simulink model "gm_uz_dac_spi_interface"  (R2023a)
settings: Solver=FixedStepDiscrete  StartTime=0.0  StopTime=2000/100e6  RelTol=1e-3
libraries: hdlsllib x152, simulink x3
settings Model: Creator=ts  LastModifiedBy=ts
settings SolverCC: AlgebraicLoopSolver=TrustRegion
settings DataIOCC: LimitDataPoints=on  SaveOutput=off  SaveTime=off
settings OptimizationCC: BlockReduction=off  ConditionallyExecuteInputs=off  DefaultParameterBehavior=Inlined  LifeSpan=inf
settings DebuggingCC: AlgebraicLoopMsg=error  InheritedTsInSrcMsg=none  SingleTaskRateTransMsg=error  UnconnectedInputMsg=warning  UnconnectedOutputMsg=warning  UnconnectedLineMsg=warning  AllowSymbolicDim=off  StrictBusMsg=ErrorOnBusTreatedAsVector  SFUnexpectedBacktrackingDiag=warning  SFNoUnconditionalDefaultTransitionDiag=warning  SFExecutionAtInitializationDiag=none  ArithmeticOperatorsInVariantConditions=warning
settings HardwareCC: ProdBitPerPointer=32  ProdBitPerSizeT=32  ProdBitPerPtrDiffT=32  ProdLargestAtomicFloat=None  ProdIntDivRoundTo=Undefined  ProdEndianess=Unspecified  ProdWordSize=32  ProdHWDeviceType=ASIC/FPGA->ASIC/FPGA  ProdEqTarget=off
settings ModelReferenceCC: EnableRefExpFcnMdlSchedulingChecks=on
settings SFSimCC: SimUseLocalCustomCode=off  CustomCodeUndefinedFunction=UseInterfaceOnly
settings RTWCC: RTWUseLocalCustomCode=off
settings CodeAppCC: StateflowObjectComments=on
settings GRTTargetCC: TargetLangStandard=C89/C90 (ANSI)
settings ConfigComp: CovScope=ReferencedModels  CovMetricSettings=dw  CovSaveCumulativeToWorkspaceVar=on  CovSaveSingleToWorkspaceVar=on  CovExternalEMLEnable=off  CovSFcnEnable=off

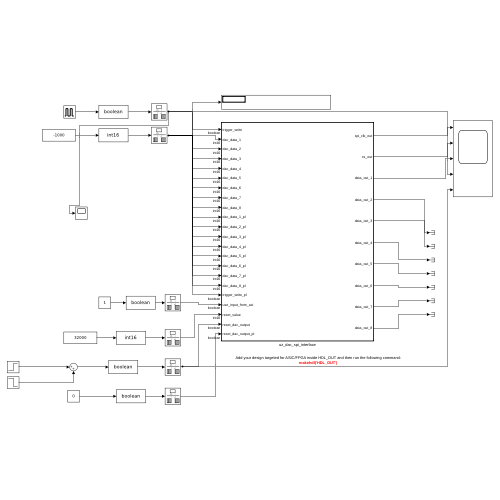
[thumbnail: Simulink's stored preview of the top-level diagram]
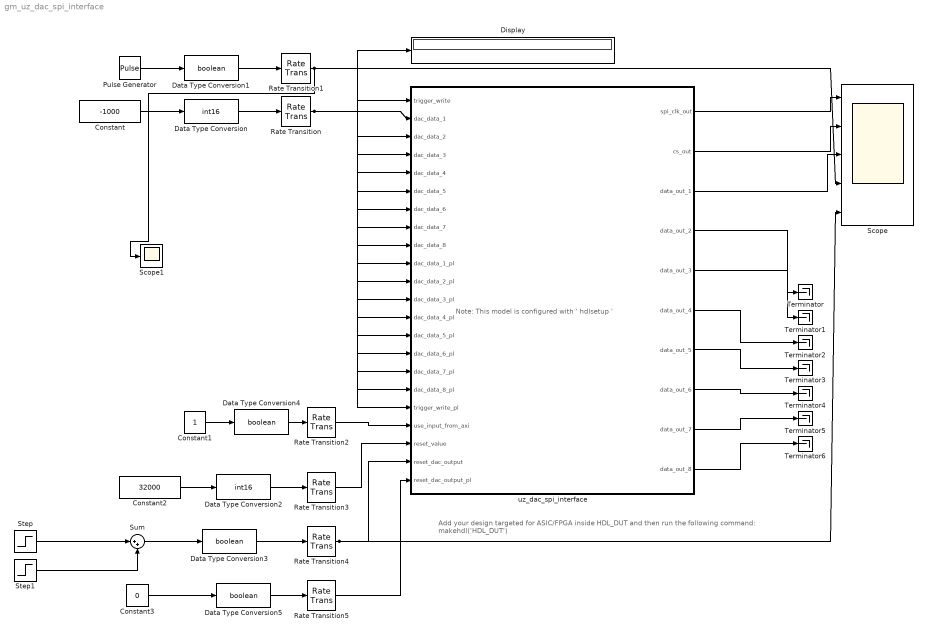
== system gm_uz_dac_spi_interface ==
  note: Add your design targeted for ASIC/FPGA inside HDL_DUT and then run the following command:
      | makehdl('HDL_DUT')
  note: Note: This model is configured with ' hdlsetup '
  Constant : Constant  Value=-1000  OutDataTypeStr=int16  SampleTime=1/100e6
  Constant1 : Constant
  Constant2 : Constant  Value=32000  OutDataTypeStr=int16  SampleTime=1/100e6
  Constant3 : Constant  Value=0
  Data Type Conversion : DataTypeConversion  OutDataTypeStr=int16  SaturateOnIntegerOverflow=off  RndMeth=Floor
  Data Type Conversion{1,3..5} (4 alike) : DataTypeConversion  OutDataTypeStr=boolean  SaturateOnIntegerOverflow=off  RndMeth=Floor
  Data Type Conversion2 : DataTypeConversion  OutDataTypeStr=int16  SaturateOnIntegerOverflow=off  RndMeth=Floor
  Display : Display
      settings: Format=binary (Stored Integer)
  Pulse Generator : DiscretePulseGenerator  PulseType=Time based  Period=200/100e6  PulseWidth=10
  Rate Transition{,1..5} (6 alike) : RateTransition  OutPortSampleTime=1/100e6
  Scope : Scope  NumInputPorts=5
  Scope1 : Scope
  Step : Step  Time=280/100e6  SampleTime=1/100e6  VectorParams1D=off
  Step1 : Step  Time=800/100e6  After=-1  SampleTime=1/100e6
  Sum : Sum  Inputs=|++
  Terminator{,1..6} (7 alike) : Terminator
  uz_dac_spi_interface : Subsystem  TreatAsAtomicUnit=on
  wires:
  Sum/1 -> Data Type Conversion3/1
  Step1/1 -> Sum/2
  Step/1 -> Sum/1
  Rate Transition4/1 -> uz_dac_spi_interface/21(reset_dac_output), Scope/5
  Data Type Conversion5/1 -> Rate Transition5/1
  Data Type Conversion4/1 -> Rate Transition2/1
  Rate Transition5/1 -> uz_dac_spi_interface/22(reset_dac_output_pl)
  Constant3/1 -> Data Type Conversion5/1
  Data Type Conversion3/1 -> Rate Transition4/1
  Rate Transition3/1 -> uz_dac_spi_interface/20(reset_value)
  Data Type Conversion2/1 -> Rate Transition3/1
  Constant2/1 -> Data Type Conversion2/1
  uz_dac_spi_interface/10(data_out_8) -> Terminator6/1
  uz_dac_spi_interface/9(data_out_7) -> Terminator5/1
  uz_dac_spi_interface/8(data_out_6) -> Terminator4/1
  uz_dac_spi_interface/7(data_out_5) -> Terminator3/1
  uz_dac_spi_interface/6(data_out_4) -> Terminator2/1
  uz_dac_spi_interface/5(data_out_3) -> Terminator1/1
  uz_dac_spi_interface/4(data_out_2) -> Terminator/1
  Constant1/1 -> Data Type Conversion4/1
  Rate Transition2/1 -> uz_dac_spi_interface/19(use_input_from_axi)
  Pulse Generator/1 -> Data Type Conversion1/1
  Data Type Conversion1/1 -> Rate Transition1/1
  Rate Transition1/1 -> Scope1/1, uz_dac_spi_interface/18(trigger_write_pl), uz_dac_spi_interface/1(trigger_write), Scope/4
  uz_dac_spi_interface/1(spi_clk_out) -> Scope/1
  uz_dac_spi_interface/2(cs_out) -> Scope/2
  Rate Transition/1 -> uz_dac_spi_interface/2(dac_data_1), uz_dac_spi_interface/3(dac_data_2), uz_dac_spi_interface/4(dac_data_3), uz_dac_spi_interface/5(dac_data_4), uz_dac_spi_interface/6(dac_data_5), uz_dac_spi_interface/8(dac_data_7), uz_dac_spi_interface/9(dac_data_8), uz_dac_spi_interface/10(dac_data_1_pl), uz_dac_spi_interface/11(dac_data_2_pl), uz_dac_spi_interface/12(dac_data_3_pl), uz_dac_spi_interface/13(dac_data_4_pl), uz_dac_spi_interface/14(dac_data_5_pl), uz_dac_spi_interface/15(dac_data_6_pl), uz_dac_spi_interface/16(dac_data_7_pl), uz_dac_spi_interface/17(dac_data_8_pl), uz_dac_spi_interface/7(dac_data_6), Display/1
  Data Type Conversion/1 -> Rate Transition/1
  uz_dac_spi_interface/3(data_out_1) -> Scope/3
  Constant/1 -> Data Type Conversion/1

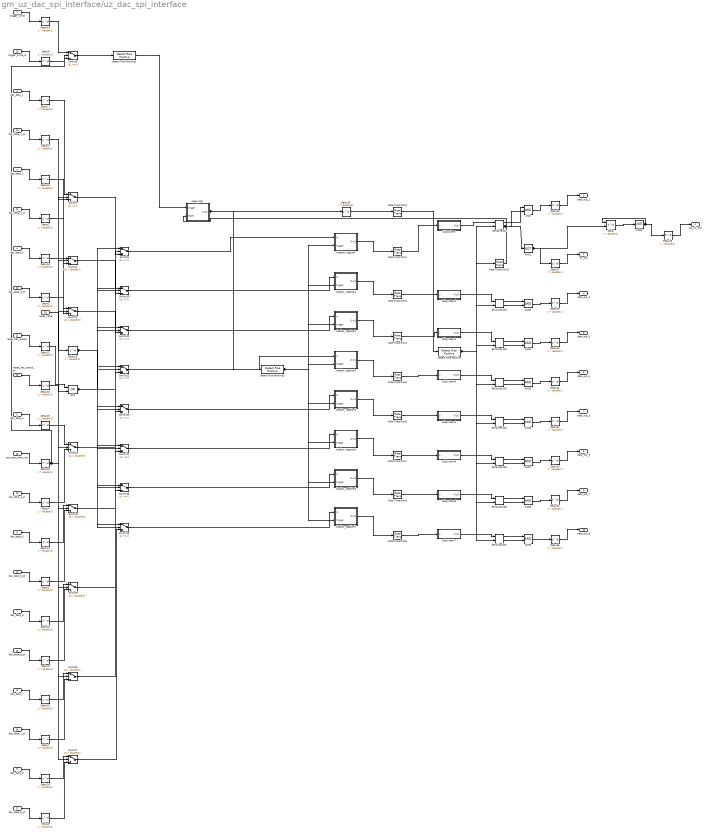
== system gm_uz_dac_spi_interface/uz_dac_spi_interface ==
  trigger_write : Inport  OutDataTypeStr=boolean  PortDimensions=1  SampleTime=1e-08
  dac_data_1 : Inport  Port=2  OutDataTypeStr=int16  PortDimensions=1  SampleTime=1e-08
  dac_data_2 : Inport  Port=3  OutDataTypeStr=int16  PortDimensions=1  SampleTime=1e-08
  dac_data_3 : Inport  Port=4  OutDataTypeStr=int16  PortDimensions=1  SampleTime=1e-08
  dac_data_4 : Inport  Port=5  OutDataTypeStr=int16  PortDimensions=1  SampleTime=1e-08
  dac_data_5 : Inport  Port=6  OutDataTypeStr=int16  PortDimensions=1  SampleTime=1e-08
  dac_data_6 : Inport  Port=7  OutDataTypeStr=int16  PortDimensions=1  SampleTime=1e-08
  dac_data_7 : Inport  Port=8  OutDataTypeStr=int16  PortDimensions=1  SampleTime=1e-08
  dac_data_8 : Inport  Port=9  OutDataTypeStr=int16  PortDimensions=1  SampleTime=1e-08
  dac_data_1_pl : Inport  Port=10  OutDataTypeStr=int16  PortDimensions=1  SampleTime=1e-08
  dac_data_2_pl : Inport  Port=11  OutDataTypeStr=int16  PortDimensions=1  SampleTime=1e-08
  dac_data_3_pl : Inport  Port=12  OutDataTypeStr=int16  PortDimensions=1  SampleTime=1e-08
  dac_data_4_pl : Inport  Port=13  OutDataTypeStr=int16  PortDimensions=1  SampleTime=1e-08
  dac_data_5_pl : Inport  Port=14  OutDataTypeStr=int16  PortDimensions=1  SampleTime=1e-08
  dac_data_6_pl : Inport  Port=15  OutDataTypeStr=int16  PortDimensions=1  SampleTime=1e-08
  dac_data_7_pl : Inport  Port=16  OutDataTypeStr=int16  PortDimensions=1  SampleTime=1e-08
  dac_data_8_pl : Inport  Port=17  OutDataTypeStr=int16  PortDimensions=1  SampleTime=1e-08
  trigger_write_pl : Inport  Port=18  OutDataTypeStr=boolean  PortDimensions=1  SampleTime=1e-08
  use_input_from_axi : Inport  Port=19  OutDataTypeStr=boolean  PortDimensions=1  SampleTime=1e-08
  reset_value : Inport  Port=20  OutDataTypeStr=int16  PortDimensions=1  SampleTime=1e-08
  reset_dac_output : Inport  Port=21  OutDataTypeStr=boolean  PortDimensions=1  SampleTime=1e-08
  reset_dac_output_pl : Inport  Port=22  OutDataTypeStr=boolean  PortDimensions=1  SampleTime=1e-08
  AND{,3..9} (8 alike) : Logic  AllPortsSameDT=off  OutDataTypeStr=boolean  SampleTime=1e-08
  AND1 : Logic  Operator=NOT  Inputs=1  AllPortsSameDT=off  OutDataTypeStr=boolean  SampleTime=1e-08
  AND2 : Logic  Operator=NOT  Inputs=1  AllPortsSameDT=off  OutDataTypeStr=boolean  SampleTime=1e-08
  Delay : Delay  DelayLength=double(1)  InitialCondition=1  ExternalReset=Level
      settings: InputPortMap=u0,r5
  Delay{1..10,12..15,17..35} (33 alike) : Delay  DelayLength=double(1)  InitialCondition=0  SampleTime=1e-08
  Detect Rise Positive : simulink/Logic and Bit Operations/Detect Rise Positive  vinit=0  OutDataTypeStr=boolean
  Detect Rise Positive1 : simulink/Logic and Bit Operations/Detect Rise Positive  vinit=0  OutDataTypeStr=boolean
  Detect Rise Positive2 : simulink/Logic and Bit Operations/Detect Rise Positive  vinit=0  OutDataTypeStr=boolean
  OR1 : Logic  Operator=OR  AllPortsSameDT=off  OutDataTypeStr=boolean  SampleTime=1e-08
  Rate Transition{1..9} (9 alike) : RateTransition  InitialCondition=double(0)  OutPortSampleTimeOpt=Multiple of input port sample time  OutPortSampleTimeMultiple=32
  Rate Transition11 : RateTransition  InitialCondition=double(0)  OutPortSampleTimeOpt=Multiple of input port sample time  OutPortSampleTimeMultiple=1/32
  Serializer1D{,1..7} (8 alike) : hdlsllib/HDL Operations/Serializer1D  Ratio=32  IdleCycles=0  validIn=on  startOut=off  validOut=on  inputDataDimensions=32  inputSampleTime=3.2e-07  inputSignalType=real
  Subsystem : Subsystem
  Subsystem1 : Subsystem
  Subsystem2 : Subsystem
  Subsystem3 : Subsystem
  Subsystem4 : Subsystem
  Subsystem5 : Subsystem
  Subsystem6 : Subsystem
  Subsystem7 : Subsystem
  Switch{,9..16} (9 alike) : Switch  Criteria=u2 ~= 0  Threshold=double(0)  OutDataTypeStr=int16  SampleTime=1e-08  SaturateOnIntegerOverflow=off  InputSameDT=off
  Switch{1..7} (7 alike) : Switch  Criteria=u2 > Threshold  Threshold=double(0)  OutDataTypeStr=int16  SampleTime=1e-08  SaturateOnIntegerOverflow=off  InputSameDT=off
  Switch8 : Switch  Criteria=u2 ~= 0  Threshold=double(0)  OutDataTypeStr=boolean  SampleTime=1e-08  SaturateOnIntegerOverflow=off  InputSameDT=off
  keep_high : Subsystem
  shadow_register : Subsystem
  shadow_register1 : Subsystem
  shadow_register2 : Subsystem
  shadow_register3 : Subsystem
  shadow_register4 : Subsystem
  shadow_register5 : Subsystem
  shadow_register6 : Subsystem
  shadow_register7 : Subsystem
  spi_clk_out : Outport  SampleTime=1e-08
  cs_out : Outport  Port=2  SampleTime=1e-08
  data_out_1 : Outport  Port=3  SampleTime=1e-08  VectorParamsAs1DForOutWhenUnconnected=off
  data_out_2 : Outport  Port=4  SampleTime=1e-08  VectorParamsAs1DForOutWhenUnconnected=off
  data_out_3 : Outport  Port=5  SampleTime=1e-08  VectorParamsAs1DForOutWhenUnconnected=off
  data_out_4 : Outport  Port=6  SampleTime=1e-08  VectorParamsAs1DForOutWhenUnconnected=off
  data_out_5 : Outport  Port=7  SampleTime=1e-08  VectorParamsAs1DForOutWhenUnconnected=off
  data_out_6 : Outport  Port=8  SampleTime=1e-08  VectorParamsAs1DForOutWhenUnconnected=off
  data_out_7 : Outport  Port=9  SampleTime=1e-08  VectorParamsAs1DForOutWhenUnconnected=off
  data_out_8 : Outport  Port=10  SampleTime=1e-08  VectorParamsAs1DForOutWhenUnconnected=off
  wires:
  trigger_write/1 -> Delay14/1
  dac_data_1/1 -> Delay17/1
  dac_data_2/1 -> Delay19/1
  dac_data_3/1 -> Delay18/1
  dac_data_4/1 -> Delay20/1
  dac_data_5/1 -> Delay21/1
  dac_data_6/1 -> Delay22/1
  dac_data_7/1 -> Delay23/1
  dac_data_8/1 -> Delay24/1
  dac_data_1_pl/1 -> Delay1/1
  dac_data_2_pl/1 -> Delay2/1
  dac_data_3_pl/1 -> Delay3/1
  dac_data_4_pl/1 -> Delay4/1
  dac_data_5_pl/1 -> Delay5/1
  dac_data_6_pl/1 -> Delay6/1
  dac_data_7_pl/1 -> Delay7/1
  dac_data_8_pl/1 -> Delay8/1
  trigger_write_pl/1 -> Delay9/1
  use_input_from_axi/1 -> Delay15/1
  reset_value/1 -> Delay13/1
  reset_dac_output/1 -> Delay12/1
  reset_dac_output_pl/1 -> Delay10/1
  AND/1 -> Delay28/1
  AND1/1 -> Delay27/1, Delay/2
  AND2/1 -> Delay26/1, Delay/1
  AND3/1 -> Delay29/1
  AND4/1 -> Delay30/1
  AND5/1 -> Delay31/1
  AND6/1 -> Delay32/1
  AND7/1 -> Delay33/1
  AND8/1 -> Delay34/1
  AND9/1 -> Delay35/1
  Delay/1 -> AND2/1
  Delay1/1 -> Switch/3
  Delay10/1 -> OR1/2
  Delay12/1 -> OR1/1
  Delay13/1 -> Switch9/1, Switch16/1, Switch15/1, Switch14/1, Switch13/1, Switch12/1, Switch11/1, Switch10/1
  Delay14/1 -> Switch8/1
  Delay15/1 -> Switch8/2, Switch7/2, Switch6/2, Switch5/2, Switch4/2, Switch3/2, Switch2/2, Switch1/2, Switch/2
  Delay17/1 -> Switch/1
  Delay18/1 -> Switch2/1
  Delay19/1 -> Switch1/1
  Delay2/1 -> Switch1/3
  Delay20/1 -> Switch3/1
  Delay21/1 -> Switch4/1
  Delay22/1 -> Switch5/1
  Delay23/1 -> Switch6/1
  Delay24/1 -> Switch7/1
  Delay25/1 -> Rate Transition2/1
  Delay26/1 -> spi_clk_out/1
  Delay27/1 -> cs_out/1
  Delay28/1 -> data_out_1/1
  Delay29/1 -> data_out_2/1
  Delay3/1 -> Switch2/3
  Delay30/1 -> data_out_3/1
  Delay31/1 -> data_out_4/1
  Delay32/1 -> data_out_5/1
  Delay33/1 -> data_out_6/1
  Delay34/1 -> data_out_7/1
  Delay35/1 -> data_out_8/1
  Delay4/1 -> Switch3/3
  Delay5/1 -> Switch4/3
  Delay6/1 -> Switch5/3
  Delay7/1 -> Switch6/3
  Delay8/1 -> Switch7/3
  Delay9/1 -> Switch8/3
  Detect Rise Positive/1 -> Serializer1D7/2, Serializer1D6/2, Serializer1D5/2, Serializer1D4/2, Serializer1D3/2, Serializer1D2/2, Serializer1D1/2, Serializer1D/2, Rate Transition11/1
  Detect Rise Positive1/1 -> keep_high/1(trigger)
  Detect Rise Positive2/1 -> shadow_register7/2(trigger), shadow_register6/2(trigger), shadow_register5/2(trigger), shadow_register4/2(trigger), shadow_register3/2(trigger), shadow_register2/2(trigger), shadow_register1/2(trigger), shadow_register/2(trigger)
  OR1/1 -> Switch9/2, Switch16/2, Switch15/2, Switch14/2, Switch13/2, Switch12/2, Switch11/2, Switch10/2
  Rate Transition1/1 -> Subsystem/1(u)
  Rate Transition11/1 -> keep_high/2(reset)
  Rate Transition2/1 -> Detect Rise Positive/1
  Rate Transition3/1 -> Subsystem1/1(u)
  Rate Transition4/1 -> Subsystem2/1(u)
  Rate Transition5/1 -> Subsystem3/1(u)
  Rate Transition6/1 -> Subsystem4/1(u)
  Rate Transition7/1 -> Subsystem5/1(u)
  Rate Transition8/1 -> Subsystem6/1(u)
  Rate Transition9/1 -> Subsystem7/1(u)
  Serializer1D/1 -> AND/1
  Serializer1D/2 -> AND1/1, AND/2
  Serializer1D1/1 -> AND3/1
  Serializer1D1/2 -> AND3/2
  Serializer1D2/1 -> AND4/1
  Serializer1D2/2 -> AND4/2
  Serializer1D3/1 -> AND5/1
  Serializer1D3/2 -> AND5/2
  Serializer1D4/1 -> AND6/1
  Serializer1D4/2 -> AND6/2
  Serializer1D5/1 -> AND7/1
  Serializer1D5/2 -> AND7/2
  Serializer1D6/1 -> AND8/1
  Serializer1D6/2 -> AND8/2
  Serializer1D7/1 -> AND9/1
  Serializer1D7/2 -> AND9/2
  Subsystem/1(Out1) -> Serializer1D/1
  Subsystem1/1(Out1) -> Serializer1D1/1
  Subsystem2/1(Out1) -> Serializer1D2/1
  Subsystem3/1(Out1) -> Serializer1D3/1
  Subsystem4/1(Out1) -> Serializer1D4/1
  Subsystem5/1(Out1) -> Serializer1D5/1
  Subsystem6/1(Out1) -> Serializer1D6/1
  Subsystem7/1(Out1) -> Serializer1D7/1
  Switch/1 -> Switch9/3
  Switch1/1 -> Switch10/3
  Switch10/1 -> shadow_register1/1(In)
  Switch11/1 -> shadow_register2/1(In)
  Switch12/1 -> shadow_register3/1(In)
  Switch13/1 -> shadow_register4/1(In)
  Switch14/1 -> shadow_register5/1(In)
  Switch15/1 -> shadow_register6/1(In)
  Switch16/1 -> shadow_register7/1(In)
  Switch2/1 -> Switch11/3
  Switch3/1 -> Switch12/3
  Switch4/1 -> Switch13/3
  Switch5/1 -> Switch14/3
  Switch6/1 -> Switch15/3
  Switch7/1 -> Switch16/3
  Switch8/1 -> Detect Rise Positive1/1
  Switch9/1 -> shadow_register/1(In)
  keep_high/1(Out1) -> Delay25/1, Detect Rise Positive2/1
  shadow_register/1(Out1) -> Rate Transition1/1
  shadow_register1/1(Out1) -> Rate Transition3/1
  shadow_register2/1(Out1) -> Rate Transition4/1
  shadow_register3/1(Out1) -> Rate Transition5/1
  shadow_register4/1(Out1) -> Rate Transition6/1
  shadow_register5/1(Out1) -> Rate Transition7/1
  shadow_register6/1(Out1) -> Rate Transition8/1
  shadow_register7/1(Out1) -> Rate Transition9/1

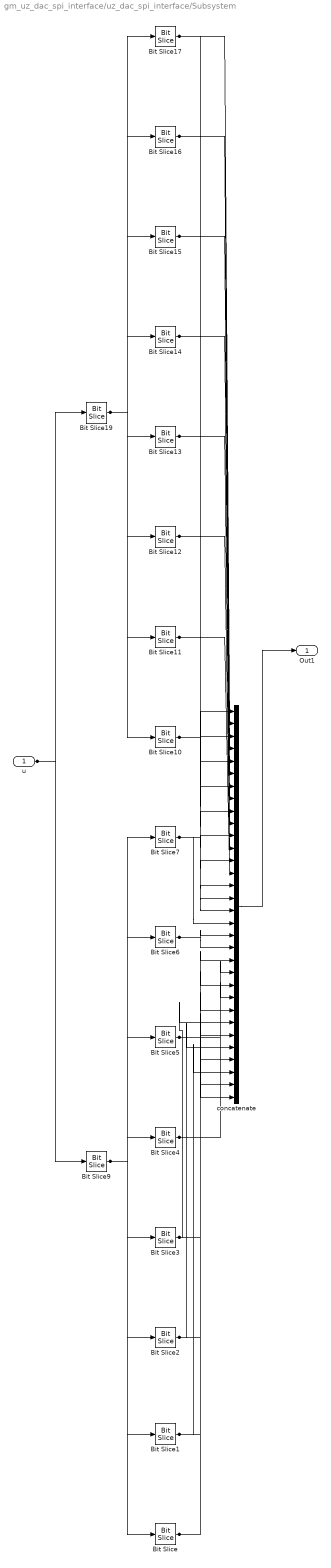
== system gm_uz_dac_spi_interface/uz_dac_spi_interface/Subsystem ==
  u : Inport  OutDataTypeStr=int16  PortDimensions=1  SampleTime=3.2e-07
  Bit Slice : hdlsllib/Logic and Bit Operations/Bit Slice  lidx=double(0)  ridx=double(0)
  Bit Slice1 : hdlsllib/Logic and Bit Operations/Bit Slice  lidx=double(1)  ridx=double(1)
  Bit Slice10 : hdlsllib/Logic and Bit Operations/Bit Slice  lidx=double(0)  ridx=double(0)
  Bit Slice11 : hdlsllib/Logic and Bit Operations/Bit Slice  lidx=double(1)  ridx=double(1)
  Bit Slice12 : hdlsllib/Logic and Bit Operations/Bit Slice  lidx=double(2)  ridx=double(2)
  Bit Slice13 : hdlsllib/Logic and Bit Operations/Bit Slice  lidx=double(3)  ridx=double(3)
  Bit Slice14 : hdlsllib/Logic and Bit Operations/Bit Slice  lidx=double(4)  ridx=double(4)
  Bit Slice15 : hdlsllib/Logic and Bit Operations/Bit Slice  lidx=double(5)  ridx=double(5)
  Bit Slice16 : hdlsllib/Logic and Bit Operations/Bit Slice  lidx=double(6)  ridx=double(6)
  Bit Slice17 : hdlsllib/Logic and Bit Operations/Bit Slice  lidx=double(7)  ridx=double(7)
  Bit Slice19 : hdlsllib/Logic and Bit Operations/Bit Slice  lidx=double(15)  ridx=double(8)
  Bit Slice2 : hdlsllib/Logic and Bit Operations/Bit Slice  lidx=double(2)  ridx=double(2)
  Bit Slice3 : hdlsllib/Logic and Bit Operations/Bit Slice  lidx=double(3)  ridx=double(3)
  Bit Slice4 : hdlsllib/Logic and Bit Operations/Bit Slice  lidx=double(4)  ridx=double(4)
  Bit Slice5 : hdlsllib/Logic and Bit Operations/Bit Slice  lidx=double(5)  ridx=double(5)
  Bit Slice6 : hdlsllib/Logic and Bit Operations/Bit Slice  lidx=double(6)  ridx=double(6)
  Bit Slice7 : hdlsllib/Logic and Bit Operations/Bit Slice  lidx=double(7)  ridx=double(7)
  Bit Slice9 : hdlsllib/Logic and Bit Operations/Bit Slice  lidx=double(7)  ridx=double(0)
  concatenate : Concatenate  NumInputs=32
  Out1 : Outport  SampleTime=3.2e-07
  wires:
  u/1 -> Bit Slice9/1, Bit Slice19/1
  Bit Slice/1 -> concatenate/32, concatenate/31
  Bit Slice1/1 -> concatenate/30, concatenate/29
  Bit Slice10/1 -> concatenate/16, concatenate/15
  Bit Slice11/1 -> concatenate/14, concatenate/13
  Bit Slice12/1 -> concatenate/12, concatenate/11
  Bit Slice13/1 -> concatenate/10, concatenate/9
  Bit Slice14/1 -> concatenate/8, concatenate/7
  Bit Slice15/1 -> concatenate/6, concatenate/5
  Bit Slice16/1 -> concatenate/4, concatenate/3
  Bit Slice17/1 -> concatenate/2, concatenate/1
  Bit Slice19/1 -> Bit Slice17/1, Bit Slice16/1, Bit Slice15/1, Bit Slice14/1, Bit Slice13/1, Bit Slice12/1, Bit Slice11/1, Bit Slice10/1
  Bit Slice2/1 -> concatenate/28, concatenate/27
  Bit Slice3/1 -> concatenate/26, concatenate/25
  Bit Slice4/1 -> concatenate/24, concatenate/23
  Bit Slice5/1 -> concatenate/22, concatenate/21
  Bit Slice6/1 -> concatenate/20, concatenate/19
  Bit Slice7/1 -> concatenate/18, concatenate/17
  Bit Slice9/1 -> Bit Slice7/1, Bit Slice6/1, Bit Slice5/1, Bit Slice4/1, Bit Slice3/1, Bit Slice2/1, Bit Slice1/1, Bit Slice/1
  concatenate/1 -> Out1/1

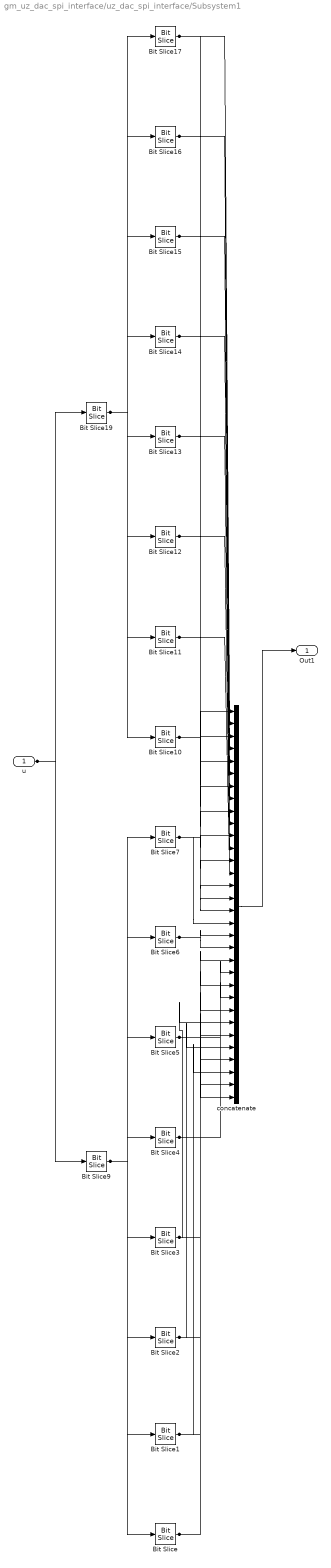
== system gm_uz_dac_spi_interface/uz_dac_spi_interface/Subsystem1 ==
  u : Inport  OutDataTypeStr=int16  PortDimensions=1  SampleTime=3.2e-07
  Bit Slice : hdlsllib/Logic and Bit Operations/Bit Slice  lidx=double(0)  ridx=double(0)
  Bit Slice1 : hdlsllib/Logic and Bit Operations/Bit Slice  lidx=double(1)  ridx=double(1)
  Bit Slice10 : hdlsllib/Logic and Bit Operations/Bit Slice  lidx=double(0)  ridx=double(0)
  Bit Slice11 : hdlsllib/Logic and Bit Operations/Bit Slice  lidx=double(1)  ridx=double(1)
  Bit Slice12 : hdlsllib/Logic and Bit Operations/Bit Slice  lidx=double(2)  ridx=double(2)
  Bit Slice13 : hdlsllib/Logic and Bit Operations/Bit Slice  lidx=double(3)  ridx=double(3)
  Bit Slice14 : hdlsllib/Logic and Bit Operations/Bit Slice  lidx=double(4)  ridx=double(4)
  Bit Slice15 : hdlsllib/Logic and Bit Operations/Bit Slice  lidx=double(5)  ridx=double(5)
  Bit Slice16 : hdlsllib/Logic and Bit Operations/Bit Slice  lidx=double(6)  ridx=double(6)
  Bit Slice17 : hdlsllib/Logic and Bit Operations/Bit Slice  lidx=double(7)  ridx=double(7)
  Bit Slice19 : hdlsllib/Logic and Bit Operations/Bit Slice  lidx=double(15)  ridx=double(8)
  Bit Slice2 : hdlsllib/Logic and Bit Operations/Bit Slice  lidx=double(2)  ridx=double(2)
  Bit Slice3 : hdlsllib/Logic and Bit Operations/Bit Slice  lidx=double(3)  ridx=double(3)
  Bit Slice4 : hdlsllib/Logic and Bit Operations/Bit Slice  lidx=double(4)  ridx=double(4)
  Bit Slice5 : hdlsllib/Logic and Bit Operations/Bit Slice  lidx=double(5)  ridx=double(5)
  Bit Slice6 : hdlsllib/Logic and Bit Operations/Bit Slice  lidx=double(6)  ridx=double(6)
  Bit Slice7 : hdlsllib/Logic and Bit Operations/Bit Slice  lidx=double(7)  ridx=double(7)
  Bit Slice9 : hdlsllib/Logic and Bit Operations/Bit Slice  lidx=double(7)  ridx=double(0)
  concatenate : Concatenate  NumInputs=32
  Out1 : Outport  SampleTime=3.2e-07
  wires:
  u/1 -> Bit Slice9/1, Bit Slice19/1
  Bit Slice/1 -> concatenate/32, concatenate/31
  Bit Slice1/1 -> concatenate/30, concatenate/29
  Bit Slice10/1 -> concatenate/16, concatenate/15
  Bit Slice11/1 -> concatenate/14, concatenate/13
  Bit Slice12/1 -> concatenate/12, concatenate/11
  Bit Slice13/1 -> concatenate/10, concatenate/9
  Bit Slice14/1 -> concatenate/8, concatenate/7
  Bit Slice15/1 -> concatenate/6, concatenate/5
  Bit Slice16/1 -> concatenate/4, concatenate/3
  Bit Slice17/1 -> concatenate/2, concatenate/1
  Bit Slice19/1 -> Bit Slice17/1, Bit Slice16/1, Bit Slice15/1, Bit Slice14/1, Bit Slice13/1, Bit Slice12/1, Bit Slice11/1, Bit Slice10/1
  Bit Slice2/1 -> concatenate/28, concatenate/27
  Bit Slice3/1 -> concatenate/26, concatenate/25
  Bit Slice4/1 -> concatenate/24, concatenate/23
  Bit Slice5/1 -> concatenate/22, concatenate/21
  Bit Slice6/1 -> concatenate/20, concatenate/19
  Bit Slice7/1 -> concatenate/18, concatenate/17
  Bit Slice9/1 -> Bit Slice7/1, Bit Slice6/1, Bit Slice5/1, Bit Slice4/1, Bit Slice3/1, Bit Slice2/1, Bit Slice1/1, Bit Slice/1
  concatenate/1 -> Out1/1

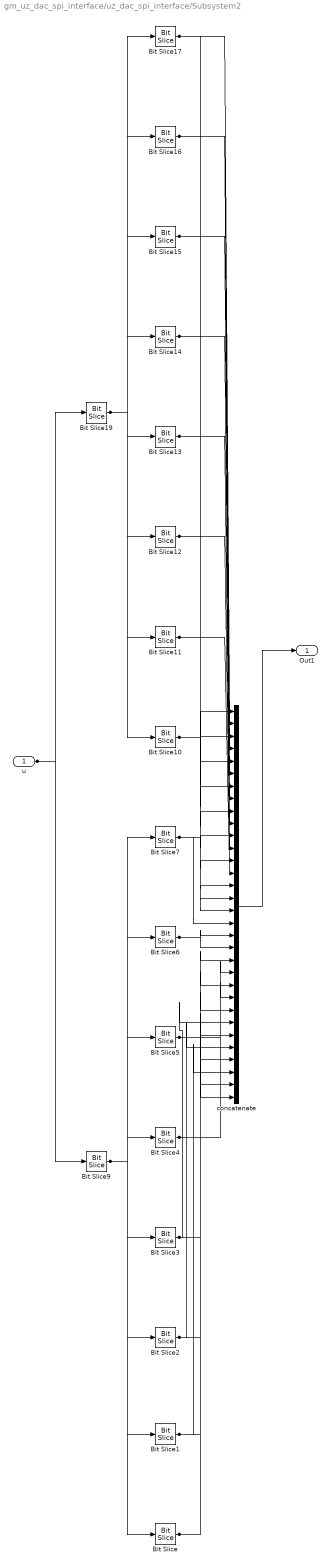
== system gm_uz_dac_spi_interface/uz_dac_spi_interface/Subsystem2 ==
  u : Inport  OutDataTypeStr=int16  PortDimensions=1  SampleTime=3.2e-07
  Bit Slice : hdlsllib/Logic and Bit Operations/Bit Slice  lidx=double(0)  ridx=double(0)
  Bit Slice1 : hdlsllib/Logic and Bit Operations/Bit Slice  lidx=double(1)  ridx=double(1)
  Bit Slice10 : hdlsllib/Logic and Bit Operations/Bit Slice  lidx=double(0)  ridx=double(0)
  Bit Slice11 : hdlsllib/Logic and Bit Operations/Bit Slice  lidx=double(1)  ridx=double(1)
  Bit Slice12 : hdlsllib/Logic and Bit Operations/Bit Slice  lidx=double(2)  ridx=double(2)
  Bit Slice13 : hdlsllib/Logic and Bit Operations/Bit Slice  lidx=double(3)  ridx=double(3)
  Bit Slice14 : hdlsllib/Logic and Bit Operations/Bit Slice  lidx=double(4)  ridx=double(4)
  Bit Slice15 : hdlsllib/Logic and Bit Operations/Bit Slice  lidx=double(5)  ridx=double(5)
  Bit Slice16 : hdlsllib/Logic and Bit Operations/Bit Slice  lidx=double(6)  ridx=double(6)
  Bit Slice17 : hdlsllib/Logic and Bit Operations/Bit Slice  lidx=double(7)  ridx=double(7)
  Bit Slice19 : hdlsllib/Logic and Bit Operations/Bit Slice  lidx=double(15)  ridx=double(8)
  Bit Slice2 : hdlsllib/Logic and Bit Operations/Bit Slice  lidx=double(2)  ridx=double(2)
  Bit Slice3 : hdlsllib/Logic and Bit Operations/Bit Slice  lidx=double(3)  ridx=double(3)
  Bit Slice4 : hdlsllib/Logic and Bit Operations/Bit Slice  lidx=double(4)  ridx=double(4)
  Bit Slice5 : hdlsllib/Logic and Bit Operations/Bit Slice  lidx=double(5)  ridx=double(5)
  Bit Slice6 : hdlsllib/Logic and Bit Operations/Bit Slice  lidx=double(6)  ridx=double(6)
  Bit Slice7 : hdlsllib/Logic and Bit Operations/Bit Slice  lidx=double(7)  ridx=double(7)
  Bit Slice9 : hdlsllib/Logic and Bit Operations/Bit Slice  lidx=double(7)  ridx=double(0)
  concatenate : Concatenate  NumInputs=32
  Out1 : Outport  SampleTime=3.2e-07
  wires:
  u/1 -> Bit Slice9/1, Bit Slice19/1
  Bit Slice/1 -> concatenate/32, concatenate/31
  Bit Slice1/1 -> concatenate/30, concatenate/29
  Bit Slice10/1 -> concatenate/16, concatenate/15
  Bit Slice11/1 -> concatenate/14, concatenate/13
  Bit Slice12/1 -> concatenate/12, concatenate/11
  Bit Slice13/1 -> concatenate/10, concatenate/9
  Bit Slice14/1 -> concatenate/8, concatenate/7
  Bit Slice15/1 -> concatenate/6, concatenate/5
  Bit Slice16/1 -> concatenate/4, concatenate/3
  Bit Slice17/1 -> concatenate/2, concatenate/1
  Bit Slice19/1 -> Bit Slice17/1, Bit Slice16/1, Bit Slice15/1, Bit Slice14/1, Bit Slice13/1, Bit Slice12/1, Bit Slice11/1, Bit Slice10/1
  Bit Slice2/1 -> concatenate/28, concatenate/27
  Bit Slice3/1 -> concatenate/26, concatenate/25
  Bit Slice4/1 -> concatenate/24, concatenate/23
  Bit Slice5/1 -> concatenate/22, concatenate/21
  Bit Slice6/1 -> concatenate/20, concatenate/19
  Bit Slice7/1 -> concatenate/18, concatenate/17
  Bit Slice9/1 -> Bit Slice7/1, Bit Slice6/1, Bit Slice5/1, Bit Slice4/1, Bit Slice3/1, Bit Slice2/1, Bit Slice1/1, Bit Slice/1
  concatenate/1 -> Out1/1

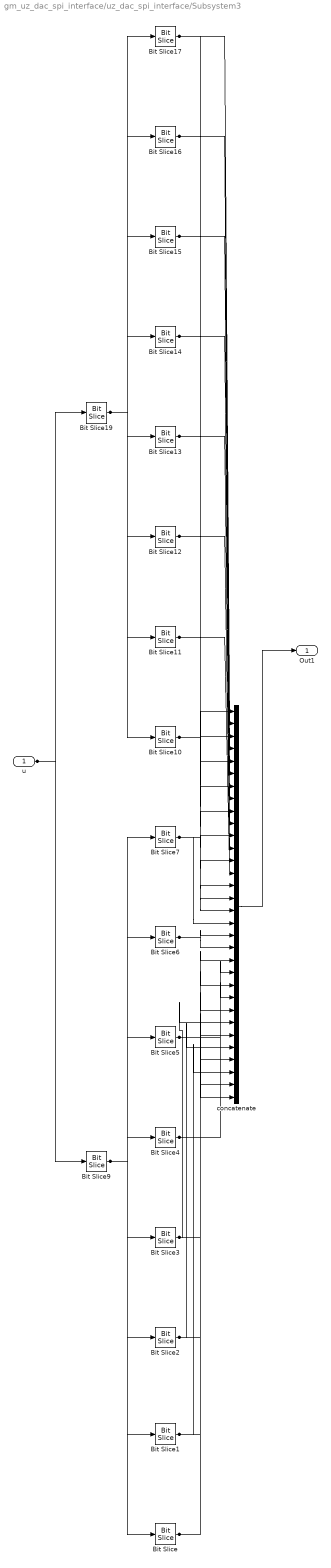
== system gm_uz_dac_spi_interface/uz_dac_spi_interface/Subsystem3 ==
  u : Inport  OutDataTypeStr=int16  PortDimensions=1  SampleTime=3.2e-07
  Bit Slice : hdlsllib/Logic and Bit Operations/Bit Slice  lidx=double(0)  ridx=double(0)
  Bit Slice1 : hdlsllib/Logic and Bit Operations/Bit Slice  lidx=double(1)  ridx=double(1)
  Bit Slice10 : hdlsllib/Logic and Bit Operations/Bit Slice  lidx=double(0)  ridx=double(0)
  Bit Slice11 : hdlsllib/Logic and Bit Operations/Bit Slice  lidx=double(1)  ridx=double(1)
  Bit Slice12 : hdlsllib/Logic and Bit Operations/Bit Slice  lidx=double(2)  ridx=double(2)
  Bit Slice13 : hdlsllib/Logic and Bit Operations/Bit Slice  lidx=double(3)  ridx=double(3)
  Bit Slice14 : hdlsllib/Logic and Bit Operations/Bit Slice  lidx=double(4)  ridx=double(4)
  Bit Slice15 : hdlsllib/Logic and Bit Operations/Bit Slice  lidx=double(5)  ridx=double(5)
  Bit Slice16 : hdlsllib/Logic and Bit Operations/Bit Slice  lidx=double(6)  ridx=double(6)
  Bit Slice17 : hdlsllib/Logic and Bit Operations/Bit Slice  lidx=double(7)  ridx=double(7)
  Bit Slice19 : hdlsllib/Logic and Bit Operations/Bit Slice  lidx=double(15)  ridx=double(8)
  Bit Slice2 : hdlsllib/Logic and Bit Operations/Bit Slice  lidx=double(2)  ridx=double(2)
  Bit Slice3 : hdlsllib/Logic and Bit Operations/Bit Slice  lidx=double(3)  ridx=double(3)
  Bit Slice4 : hdlsllib/Logic and Bit Operations/Bit Slice  lidx=double(4)  ridx=double(4)
  Bit Slice5 : hdlsllib/Logic and Bit Operations/Bit Slice  lidx=double(5)  ridx=double(5)
  Bit Slice6 : hdlsllib/Logic and Bit Operations/Bit Slice  lidx=double(6)  ridx=double(6)
  Bit Slice7 : hdlsllib/Logic and Bit Operations/Bit Slice  lidx=double(7)  ridx=double(7)
  Bit Slice9 : hdlsllib/Logic and Bit Operations/Bit Slice  lidx=double(7)  ridx=double(0)
  concatenate : Concatenate  NumInputs=32
  Out1 : Outport  SampleTime=3.2e-07
  wires:
  u/1 -> Bit Slice9/1, Bit Slice19/1
  Bit Slice/1 -> concatenate/32, concatenate/31
  Bit Slice1/1 -> concatenate/30, concatenate/29
  Bit Slice10/1 -> concatenate/16, concatenate/15
  Bit Slice11/1 -> concatenate/14, concatenate/13
  Bit Slice12/1 -> concatenate/12, concatenate/11
  Bit Slice13/1 -> concatenate/10, concatenate/9
  Bit Slice14/1 -> concatenate/8, concatenate/7
  Bit Slice15/1 -> concatenate/6, concatenate/5
  Bit Slice16/1 -> concatenate/4, concatenate/3
  Bit Slice17/1 -> concatenate/2, concatenate/1
  Bit Slice19/1 -> Bit Slice17/1, Bit Slice16/1, Bit Slice15/1, Bit Slice14/1, Bit Slice13/1, Bit Slice12/1, Bit Slice11/1, Bit Slice10/1
  Bit Slice2/1 -> concatenate/28, concatenate/27
  Bit Slice3/1 -> concatenate/26, concatenate/25
  Bit Slice4/1 -> concatenate/24, concatenate/23
  Bit Slice5/1 -> concatenate/22, concatenate/21
  Bit Slice6/1 -> concatenate/20, concatenate/19
  Bit Slice7/1 -> concatenate/18, concatenate/17
  Bit Slice9/1 -> Bit Slice7/1, Bit Slice6/1, Bit Slice5/1, Bit Slice4/1, Bit Slice3/1, Bit Slice2/1, Bit Slice1/1, Bit Slice/1
  concatenate/1 -> Out1/1

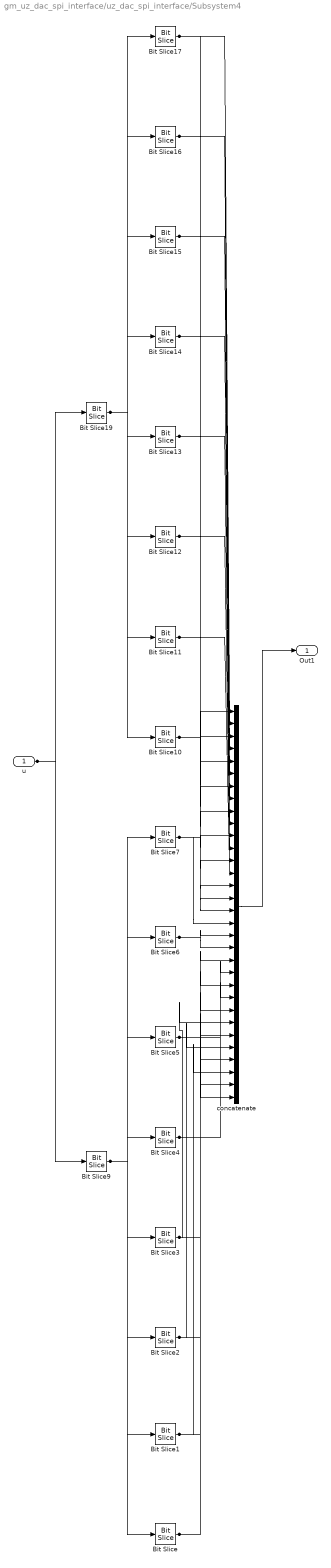
== system gm_uz_dac_spi_interface/uz_dac_spi_interface/Subsystem4 ==
  u : Inport  OutDataTypeStr=int16  PortDimensions=1  SampleTime=3.2e-07
  Bit Slice : hdlsllib/Logic and Bit Operations/Bit Slice  lidx=double(0)  ridx=double(0)
  Bit Slice1 : hdlsllib/Logic and Bit Operations/Bit Slice  lidx=double(1)  ridx=double(1)
  Bit Slice10 : hdlsllib/Logic and Bit Operations/Bit Slice  lidx=double(0)  ridx=double(0)
  Bit Slice11 : hdlsllib/Logic and Bit Operations/Bit Slice  lidx=double(1)  ridx=double(1)
  Bit Slice12 : hdlsllib/Logic and Bit Operations/Bit Slice  lidx=double(2)  ridx=double(2)
  Bit Slice13 : hdlsllib/Logic and Bit Operations/Bit Slice  lidx=double(3)  ridx=double(3)
  Bit Slice14 : hdlsllib/Logic and Bit Operations/Bit Slice  lidx=double(4)  ridx=double(4)
  Bit Slice15 : hdlsllib/Logic and Bit Operations/Bit Slice  lidx=double(5)  ridx=double(5)
  Bit Slice16 : hdlsllib/Logic and Bit Operations/Bit Slice  lidx=double(6)  ridx=double(6)
  Bit Slice17 : hdlsllib/Logic and Bit Operations/Bit Slice  lidx=double(7)  ridx=double(7)
  Bit Slice19 : hdlsllib/Logic and Bit Operations/Bit Slice  lidx=double(15)  ridx=double(8)
  Bit Slice2 : hdlsllib/Logic and Bit Operations/Bit Slice  lidx=double(2)  ridx=double(2)
  Bit Slice3 : hdlsllib/Logic and Bit Operations/Bit Slice  lidx=double(3)  ridx=double(3)
  Bit Slice4 : hdlsllib/Logic and Bit Operations/Bit Slice  lidx=double(4)  ridx=double(4)
  Bit Slice5 : hdlsllib/Logic and Bit Operations/Bit Slice  lidx=double(5)  ridx=double(5)
  Bit Slice6 : hdlsllib/Logic and Bit Operations/Bit Slice  lidx=double(6)  ridx=double(6)
  Bit Slice7 : hdlsllib/Logic and Bit Operations/Bit Slice  lidx=double(7)  ridx=double(7)
  Bit Slice9 : hdlsllib/Logic and Bit Operations/Bit Slice  lidx=double(7)  ridx=double(0)
  concatenate : Concatenate  NumInputs=32
  Out1 : Outport  SampleTime=3.2e-07
  wires:
  u/1 -> Bit Slice9/1, Bit Slice19/1
  Bit Slice/1 -> concatenate/32, concatenate/31
  Bit Slice1/1 -> concatenate/30, concatenate/29
  Bit Slice10/1 -> concatenate/16, concatenate/15
  Bit Slice11/1 -> concatenate/14, concatenate/13
  Bit Slice12/1 -> concatenate/12, concatenate/11
  Bit Slice13/1 -> concatenate/10, concatenate/9
  Bit Slice14/1 -> concatenate/8, concatenate/7
  Bit Slice15/1 -> concatenate/6, concatenate/5
  Bit Slice16/1 -> concatenate/4, concatenate/3
  Bit Slice17/1 -> concatenate/2, concatenate/1
  Bit Slice19/1 -> Bit Slice17/1, Bit Slice16/1, Bit Slice15/1, Bit Slice14/1, Bit Slice13/1, Bit Slice12/1, Bit Slice11/1, Bit Slice10/1
  Bit Slice2/1 -> concatenate/28, concatenate/27
  Bit Slice3/1 -> concatenate/26, concatenate/25
  Bit Slice4/1 -> concatenate/24, concatenate/23
  Bit Slice5/1 -> concatenate/22, concatenate/21
  Bit Slice6/1 -> concatenate/20, concatenate/19
  Bit Slice7/1 -> concatenate/18, concatenate/17
  Bit Slice9/1 -> Bit Slice7/1, Bit Slice6/1, Bit Slice5/1, Bit Slice4/1, Bit Slice3/1, Bit Slice2/1, Bit Slice1/1, Bit Slice/1
  concatenate/1 -> Out1/1

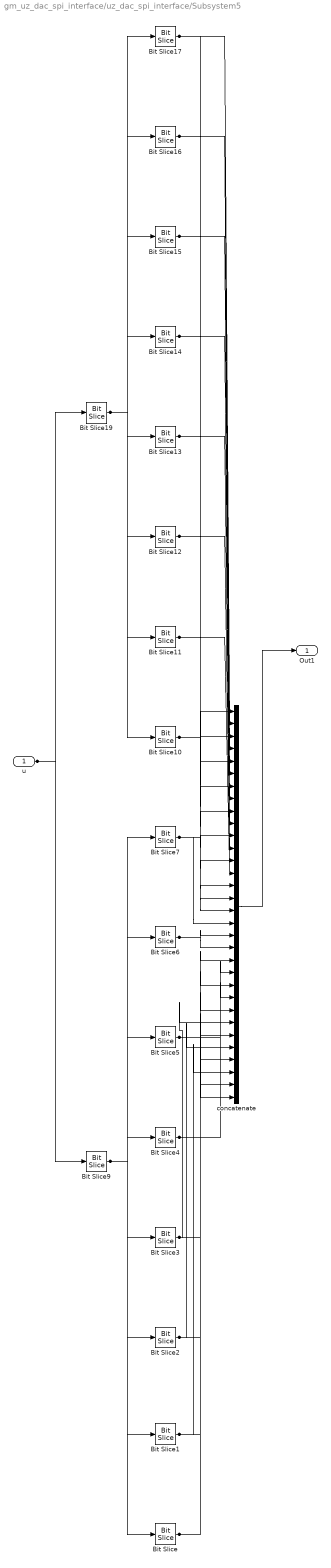
== system gm_uz_dac_spi_interface/uz_dac_spi_interface/Subsystem5 ==
  u : Inport  OutDataTypeStr=int16  PortDimensions=1  SampleTime=3.2e-07
  Bit Slice : hdlsllib/Logic and Bit Operations/Bit Slice  lidx=double(0)  ridx=double(0)
  Bit Slice1 : hdlsllib/Logic and Bit Operations/Bit Slice  lidx=double(1)  ridx=double(1)
  Bit Slice10 : hdlsllib/Logic and Bit Operations/Bit Slice  lidx=double(0)  ridx=double(0)
  Bit Slice11 : hdlsllib/Logic and Bit Operations/Bit Slice  lidx=double(1)  ridx=double(1)
  Bit Slice12 : hdlsllib/Logic and Bit Operations/Bit Slice  lidx=double(2)  ridx=double(2)
  Bit Slice13 : hdlsllib/Logic and Bit Operations/Bit Slice  lidx=double(3)  ridx=double(3)
  Bit Slice14 : hdlsllib/Logic and Bit Operations/Bit Slice  lidx=double(4)  ridx=double(4)
  Bit Slice15 : hdlsllib/Logic and Bit Operations/Bit Slice  lidx=double(5)  ridx=double(5)
  Bit Slice16 : hdlsllib/Logic and Bit Operations/Bit Slice  lidx=double(6)  ridx=double(6)
  Bit Slice17 : hdlsllib/Logic and Bit Operations/Bit Slice  lidx=double(7)  ridx=double(7)
  Bit Slice19 : hdlsllib/Logic and Bit Operations/Bit Slice  lidx=double(15)  ridx=double(8)
  Bit Slice2 : hdlsllib/Logic and Bit Operations/Bit Slice  lidx=double(2)  ridx=double(2)
  Bit Slice3 : hdlsllib/Logic and Bit Operations/Bit Slice  lidx=double(3)  ridx=double(3)
  Bit Slice4 : hdlsllib/Logic and Bit Operations/Bit Slice  lidx=double(4)  ridx=double(4)
  Bit Slice5 : hdlsllib/Logic and Bit Operations/Bit Slice  lidx=double(5)  ridx=double(5)
  Bit Slice6 : hdlsllib/Logic and Bit Operations/Bit Slice  lidx=double(6)  ridx=double(6)
  Bit Slice7 : hdlsllib/Logic and Bit Operations/Bit Slice  lidx=double(7)  ridx=double(7)
  Bit Slice9 : hdlsllib/Logic and Bit Operations/Bit Slice  lidx=double(7)  ridx=double(0)
  concatenate : Concatenate  NumInputs=32
  Out1 : Outport  SampleTime=3.2e-07
  wires:
  u/1 -> Bit Slice9/1, Bit Slice19/1
  Bit Slice/1 -> concatenate/32, concatenate/31
  Bit Slice1/1 -> concatenate/30, concatenate/29
  Bit Slice10/1 -> concatenate/16, concatenate/15
  Bit Slice11/1 -> concatenate/14, concatenate/13
  Bit Slice12/1 -> concatenate/12, concatenate/11
  Bit Slice13/1 -> concatenate/10, concatenate/9
  Bit Slice14/1 -> concatenate/8, concatenate/7
  Bit Slice15/1 -> concatenate/6, concatenate/5
  Bit Slice16/1 -> concatenate/4, concatenate/3
  Bit Slice17/1 -> concatenate/2, concatenate/1
  Bit Slice19/1 -> Bit Slice17/1, Bit Slice16/1, Bit Slice15/1, Bit Slice14/1, Bit Slice13/1, Bit Slice12/1, Bit Slice11/1, Bit Slice10/1
  Bit Slice2/1 -> concatenate/28, concatenate/27
  Bit Slice3/1 -> concatenate/26, concatenate/25
  Bit Slice4/1 -> concatenate/24, concatenate/23
  Bit Slice5/1 -> concatenate/22, concatenate/21
  Bit Slice6/1 -> concatenate/20, concatenate/19
  Bit Slice7/1 -> concatenate/18, concatenate/17
  Bit Slice9/1 -> Bit Slice7/1, Bit Slice6/1, Bit Slice5/1, Bit Slice4/1, Bit Slice3/1, Bit Slice2/1, Bit Slice1/1, Bit Slice/1
  concatenate/1 -> Out1/1

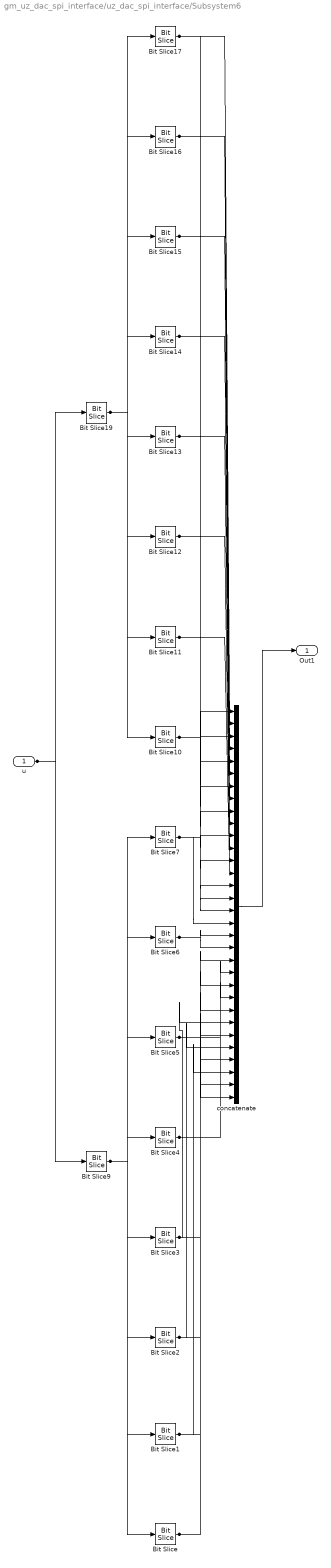
== system gm_uz_dac_spi_interface/uz_dac_spi_interface/Subsystem6 ==
  u : Inport  OutDataTypeStr=int16  PortDimensions=1  SampleTime=3.2e-07
  Bit Slice : hdlsllib/Logic and Bit Operations/Bit Slice  lidx=double(0)  ridx=double(0)
  Bit Slice1 : hdlsllib/Logic and Bit Operations/Bit Slice  lidx=double(1)  ridx=double(1)
  Bit Slice10 : hdlsllib/Logic and Bit Operations/Bit Slice  lidx=double(0)  ridx=double(0)
  Bit Slice11 : hdlsllib/Logic and Bit Operations/Bit Slice  lidx=double(1)  ridx=double(1)
  Bit Slice12 : hdlsllib/Logic and Bit Operations/Bit Slice  lidx=double(2)  ridx=double(2)
  Bit Slice13 : hdlsllib/Logic and Bit Operations/Bit Slice  lidx=double(3)  ridx=double(3)
  Bit Slice14 : hdlsllib/Logic and Bit Operations/Bit Slice  lidx=double(4)  ridx=double(4)
  Bit Slice15 : hdlsllib/Logic and Bit Operations/Bit Slice  lidx=double(5)  ridx=double(5)
  Bit Slice16 : hdlsllib/Logic and Bit Operations/Bit Slice  lidx=double(6)  ridx=double(6)
  Bit Slice17 : hdlsllib/Logic and Bit Operations/Bit Slice  lidx=double(7)  ridx=double(7)
  Bit Slice19 : hdlsllib/Logic and Bit Operations/Bit Slice  lidx=double(15)  ridx=double(8)
  Bit Slice2 : hdlsllib/Logic and Bit Operations/Bit Slice  lidx=double(2)  ridx=double(2)
  Bit Slice3 : hdlsllib/Logic and Bit Operations/Bit Slice  lidx=double(3)  ridx=double(3)
  Bit Slice4 : hdlsllib/Logic and Bit Operations/Bit Slice  lidx=double(4)  ridx=double(4)
  Bit Slice5 : hdlsllib/Logic and Bit Operations/Bit Slice  lidx=double(5)  ridx=double(5)
  Bit Slice6 : hdlsllib/Logic and Bit Operations/Bit Slice  lidx=double(6)  ridx=double(6)
  Bit Slice7 : hdlsllib/Logic and Bit Operations/Bit Slice  lidx=double(7)  ridx=double(7)
  Bit Slice9 : hdlsllib/Logic and Bit Operations/Bit Slice  lidx=double(7)  ridx=double(0)
  concatenate : Concatenate  NumInputs=32
  Out1 : Outport  SampleTime=3.2e-07
  wires:
  u/1 -> Bit Slice9/1, Bit Slice19/1
  Bit Slice/1 -> concatenate/32, concatenate/31
  Bit Slice1/1 -> concatenate/30, concatenate/29
  Bit Slice10/1 -> concatenate/16, concatenate/15
  Bit Slice11/1 -> concatenate/14, concatenate/13
  Bit Slice12/1 -> concatenate/12, concatenate/11
  Bit Slice13/1 -> concatenate/10, concatenate/9
  Bit Slice14/1 -> concatenate/8, concatenate/7
  Bit Slice15/1 -> concatenate/6, concatenate/5
  Bit Slice16/1 -> concatenate/4, concatenate/3
  Bit Slice17/1 -> concatenate/2, concatenate/1
  Bit Slice19/1 -> Bit Slice17/1, Bit Slice16/1, Bit Slice15/1, Bit Slice14/1, Bit Slice13/1, Bit Slice12/1, Bit Slice11/1, Bit Slice10/1
  Bit Slice2/1 -> concatenate/28, concatenate/27
  Bit Slice3/1 -> concatenate/26, concatenate/25
  Bit Slice4/1 -> concatenate/24, concatenate/23
  Bit Slice5/1 -> concatenate/22, concatenate/21
  Bit Slice6/1 -> concatenate/20, concatenate/19
  Bit Slice7/1 -> concatenate/18, concatenate/17
  Bit Slice9/1 -> Bit Slice7/1, Bit Slice6/1, Bit Slice5/1, Bit Slice4/1, Bit Slice3/1, Bit Slice2/1, Bit Slice1/1, Bit Slice/1
  concatenate/1 -> Out1/1

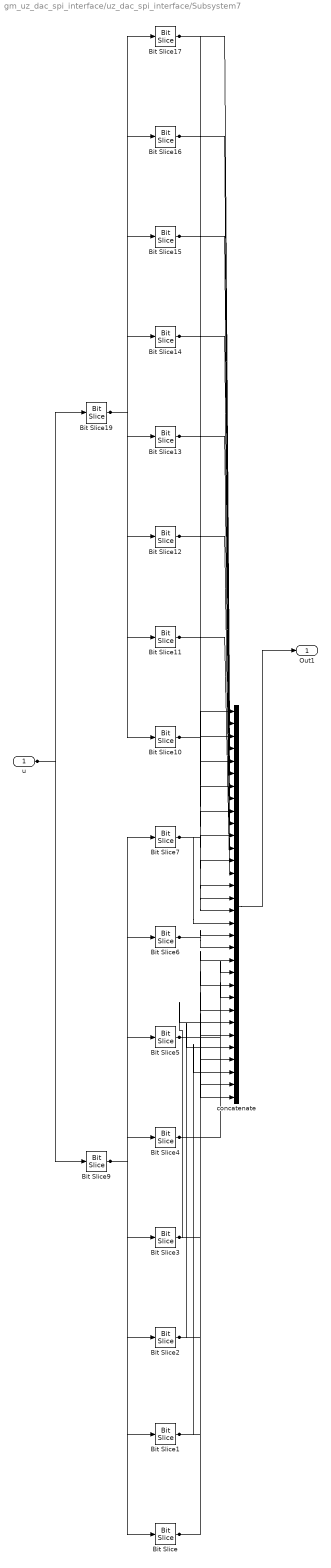
== system gm_uz_dac_spi_interface/uz_dac_spi_interface/Subsystem7 ==
  u : Inport  OutDataTypeStr=int16  PortDimensions=1  SampleTime=3.2e-07
  Bit Slice : hdlsllib/Logic and Bit Operations/Bit Slice  lidx=double(0)  ridx=double(0)
  Bit Slice1 : hdlsllib/Logic and Bit Operations/Bit Slice  lidx=double(1)  ridx=double(1)
  Bit Slice10 : hdlsllib/Logic and Bit Operations/Bit Slice  lidx=double(0)  ridx=double(0)
  Bit Slice11 : hdlsllib/Logic and Bit Operations/Bit Slice  lidx=double(1)  ridx=double(1)
  Bit Slice12 : hdlsllib/Logic and Bit Operations/Bit Slice  lidx=double(2)  ridx=double(2)
  Bit Slice13 : hdlsllib/Logic and Bit Operations/Bit Slice  lidx=double(3)  ridx=double(3)
  Bit Slice14 : hdlsllib/Logic and Bit Operations/Bit Slice  lidx=double(4)  ridx=double(4)
  Bit Slice15 : hdlsllib/Logic and Bit Operations/Bit Slice  lidx=double(5)  ridx=double(5)
  Bit Slice16 : hdlsllib/Logic and Bit Operations/Bit Slice  lidx=double(6)  ridx=double(6)
  Bit Slice17 : hdlsllib/Logic and Bit Operations/Bit Slice  lidx=double(7)  ridx=double(7)
  Bit Slice19 : hdlsllib/Logic and Bit Operations/Bit Slice  lidx=double(15)  ridx=double(8)
  Bit Slice2 : hdlsllib/Logic and Bit Operations/Bit Slice  lidx=double(2)  ridx=double(2)
  Bit Slice3 : hdlsllib/Logic and Bit Operations/Bit Slice  lidx=double(3)  ridx=double(3)
  Bit Slice4 : hdlsllib/Logic and Bit Operations/Bit Slice  lidx=double(4)  ridx=double(4)
  Bit Slice5 : hdlsllib/Logic and Bit Operations/Bit Slice  lidx=double(5)  ridx=double(5)
  Bit Slice6 : hdlsllib/Logic and Bit Operations/Bit Slice  lidx=double(6)  ridx=double(6)
  Bit Slice7 : hdlsllib/Logic and Bit Operations/Bit Slice  lidx=double(7)  ridx=double(7)
  Bit Slice9 : hdlsllib/Logic and Bit Operations/Bit Slice  lidx=double(7)  ridx=double(0)
  concatenate : Concatenate  NumInputs=32
  Out1 : Outport  SampleTime=3.2e-07
  wires:
  u/1 -> Bit Slice9/1, Bit Slice19/1
  Bit Slice/1 -> concatenate/32, concatenate/31
  Bit Slice1/1 -> concatenate/30, concatenate/29
  Bit Slice10/1 -> concatenate/16, concatenate/15
  Bit Slice11/1 -> concatenate/14, concatenate/13
  Bit Slice12/1 -> concatenate/12, concatenate/11
  Bit Slice13/1 -> concatenate/10, concatenate/9
  Bit Slice14/1 -> concatenate/8, concatenate/7
  Bit Slice15/1 -> concatenate/6, concatenate/5
  Bit Slice16/1 -> concatenate/4, concatenate/3
  Bit Slice17/1 -> concatenate/2, concatenate/1
  Bit Slice19/1 -> Bit Slice17/1, Bit Slice16/1, Bit Slice15/1, Bit Slice14/1, Bit Slice13/1, Bit Slice12/1, Bit Slice11/1, Bit Slice10/1
  Bit Slice2/1 -> concatenate/28, concatenate/27
  Bit Slice3/1 -> concatenate/26, concatenate/25
  Bit Slice4/1 -> concatenate/24, concatenate/23
  Bit Slice5/1 -> concatenate/22, concatenate/21
  Bit Slice6/1 -> concatenate/20, concatenate/19
  Bit Slice7/1 -> concatenate/18, concatenate/17
  Bit Slice9/1 -> Bit Slice7/1, Bit Slice6/1, Bit Slice5/1, Bit Slice4/1, Bit Slice3/1, Bit Slice2/1, Bit Slice1/1, Bit Slice/1
  concatenate/1 -> Out1/1

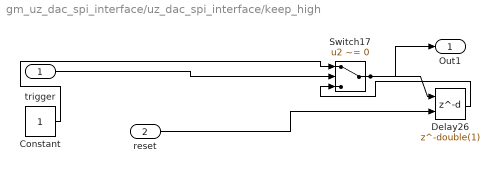
== system gm_uz_dac_spi_interface/uz_dac_spi_interface/keep_high ==
  trigger : Inport  OutDataTypeStr=boolean  PortDimensions=1  SampleTime=1e-08
  reset : Inport  Port=2  OutDataTypeStr=boolean  PortDimensions=1  SampleTime=1e-08
  Constant : Constant  OutDataTypeStr=boolean  SampleTime=1e-08
  Delay26 : Delay  DelayLength=double(1)  InitialCondition=0  ExternalReset=Level
      settings: InputPortMap=u0,r5
  Switch17 : Switch  Criteria=u2 ~= 0  Threshold=double(0)  OutDataTypeStr=int16  SampleTime=1e-08  SaturateOnIntegerOverflow=off  InputSameDT=off
  Out1 : Outport  PortDimensions=1  SampleTime=1e-08
  wires:
  trigger/1 -> Switch17/2
  reset/1 -> Delay26/2
  Constant/1 -> Switch17/1
  Delay26/1 -> Switch17/3
  Switch17/1 -> Delay26/1, Out1/1

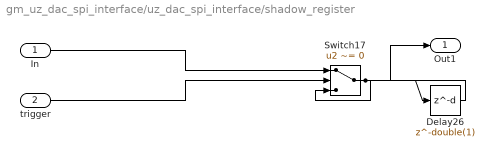
== system gm_uz_dac_spi_interface/uz_dac_spi_interface/shadow_register ==
  In : Inport  OutDataTypeStr=int16  PortDimensions=1  SampleTime=1e-08
  trigger : Inport  Port=2  OutDataTypeStr=boolean  PortDimensions=1  SampleTime=1e-08
  Delay26 : Delay  DelayLength=double(1)  InitialCondition=0  SampleTime=1e-08
  Switch17 : Switch  Criteria=u2 ~= 0  Threshold=double(0)  OutDataTypeStr=int16  SampleTime=1e-08  SaturateOnIntegerOverflow=off  InputSameDT=off
  Out1 : Outport  PortDimensions=1  SampleTime=1e-08
  wires:
  In/1 -> Switch17/1
  trigger/1 -> Switch17/2
  Delay26/1 -> Switch17/3
  Switch17/1 -> Delay26/1, Out1/1

== system gm_uz_dac_spi_interface/uz_dac_spi_interface/shadow_register1 ==
  In : Inport  OutDataTypeStr=int16  PortDimensions=1  SampleTime=1e-08
  trigger : Inport  Port=2  OutDataTypeStr=boolean  PortDimensions=1  SampleTime=1e-08
  Delay26 : Delay  DelayLength=double(1)  InitialCondition=0  SampleTime=1e-08
  Switch17 : Switch  Criteria=u2 ~= 0  Threshold=double(0)  OutDataTypeStr=int16  SampleTime=1e-08  SaturateOnIntegerOverflow=off  InputSameDT=off
  Out1 : Outport  PortDimensions=1  SampleTime=1e-08
  wires:
  In/1 -> Switch17/1
  trigger/1 -> Switch17/2
  Delay26/1 -> Switch17/3
  Switch17/1 -> Delay26/1, Out1/1

== system gm_uz_dac_spi_interface/uz_dac_spi_interface/shadow_register2 ==
  In : Inport  OutDataTypeStr=int16  PortDimensions=1  SampleTime=1e-08
  trigger : Inport  Port=2  OutDataTypeStr=boolean  PortDimensions=1  SampleTime=1e-08
  Delay26 : Delay  DelayLength=double(1)  InitialCondition=0  SampleTime=1e-08
  Switch17 : Switch  Criteria=u2 ~= 0  Threshold=double(0)  OutDataTypeStr=int16  SampleTime=1e-08  SaturateOnIntegerOverflow=off  InputSameDT=off
  Out1 : Outport  PortDimensions=1  SampleTime=1e-08
  wires:
  In/1 -> Switch17/1
  trigger/1 -> Switch17/2
  Delay26/1 -> Switch17/3
  Switch17/1 -> Delay26/1, Out1/1

== system gm_uz_dac_spi_interface/uz_dac_spi_interface/shadow_register3 ==
  In : Inport  OutDataTypeStr=int16  PortDimensions=1  SampleTime=1e-08
  trigger : Inport  Port=2  OutDataTypeStr=boolean  PortDimensions=1  SampleTime=1e-08
  Delay26 : Delay  DelayLength=double(1)  InitialCondition=0  SampleTime=1e-08
  Switch17 : Switch  Criteria=u2 ~= 0  Threshold=double(0)  OutDataTypeStr=int16  SampleTime=1e-08  SaturateOnIntegerOverflow=off  InputSameDT=off
  Out1 : Outport  PortDimensions=1  SampleTime=1e-08
  wires:
  In/1 -> Switch17/1
  trigger/1 -> Switch17/2
  Delay26/1 -> Switch17/3
  Switch17/1 -> Delay26/1, Out1/1

== system gm_uz_dac_spi_interface/uz_dac_spi_interface/shadow_register4 ==
  In : Inport  OutDataTypeStr=int16  PortDimensions=1  SampleTime=1e-08
  trigger : Inport  Port=2  OutDataTypeStr=boolean  PortDimensions=1  SampleTime=1e-08
  Delay26 : Delay  DelayLength=double(1)  InitialCondition=0  SampleTime=1e-08
  Switch17 : Switch  Criteria=u2 ~= 0  Threshold=double(0)  OutDataTypeStr=int16  SampleTime=1e-08  SaturateOnIntegerOverflow=off  InputSameDT=off
  Out1 : Outport  PortDimensions=1  SampleTime=1e-08
  wires:
  In/1 -> Switch17/1
  trigger/1 -> Switch17/2
  Delay26/1 -> Switch17/3
  Switch17/1 -> Delay26/1, Out1/1

== system gm_uz_dac_spi_interface/uz_dac_spi_interface/shadow_register5 ==
  In : Inport  OutDataTypeStr=int16  PortDimensions=1  SampleTime=1e-08
  trigger : Inport  Port=2  OutDataTypeStr=boolean  PortDimensions=1  SampleTime=1e-08
  Delay26 : Delay  DelayLength=double(1)  InitialCondition=0  SampleTime=1e-08
  Switch17 : Switch  Criteria=u2 ~= 0  Threshold=double(0)  OutDataTypeStr=int16  SampleTime=1e-08  SaturateOnIntegerOverflow=off  InputSameDT=off
  Out1 : Outport  PortDimensions=1  SampleTime=1e-08
  wires:
  In/1 -> Switch17/1
  trigger/1 -> Switch17/2
  Delay26/1 -> Switch17/3
  Switch17/1 -> Delay26/1, Out1/1

== system gm_uz_dac_spi_interface/uz_dac_spi_interface/shadow_register6 ==
  In : Inport  OutDataTypeStr=int16  PortDimensions=1  SampleTime=1e-08
  trigger : Inport  Port=2  OutDataTypeStr=boolean  PortDimensions=1  SampleTime=1e-08
  Delay26 : Delay  DelayLength=double(1)  InitialCondition=0  SampleTime=1e-08
  Switch17 : Switch  Criteria=u2 ~= 0  Threshold=double(0)  OutDataTypeStr=int16  SampleTime=1e-08  SaturateOnIntegerOverflow=off  InputSameDT=off
  Out1 : Outport  PortDimensions=1  SampleTime=1e-08
  wires:
  In/1 -> Switch17/1
  trigger/1 -> Switch17/2
  Delay26/1 -> Switch17/3
  Switch17/1 -> Delay26/1, Out1/1

== system gm_uz_dac_spi_interface/uz_dac_spi_interface/shadow_register7 ==
  In : Inport  OutDataTypeStr=int16  PortDimensions=1  SampleTime=1e-08
  trigger : Inport  Port=2  OutDataTypeStr=boolean  PortDimensions=1  SampleTime=1e-08
  Delay26 : Delay  DelayLength=double(1)  InitialCondition=0  SampleTime=1e-08
  Switch17 : Switch  Criteria=u2 ~= 0  Threshold=double(0)  OutDataTypeStr=int16  SampleTime=1e-08  SaturateOnIntegerOverflow=off  InputSameDT=off
  Out1 : Outport  PortDimensions=1  SampleTime=1e-08
  wires:
  In/1 -> Switch17/1
  trigger/1 -> Switch17/2
  Delay26/1 -> Switch17/3
  Switch17/1 -> Delay26/1, Out1/1
